simulink model "LinearSolver_System"  (R2021a)
settings: Solver=VariableStepAuto  StartTime=0.0  StopTime=1000  RelTol=1e-3
undefined symbols (not defined in the file or in its folder): AXI4, Lite
libraries: hdlBasic x415, xbsIndex_r4 x1
(part 3 of 4)

== system LinearSolver_System/Rotation4 ==
  y_in : Inport
  theta_in : Inport  Port=2
  rst : Inport  Port=3
  R_in : Inport  Port=4
  Constant3 : hdlBasic/Constant  const=0.0  gui_display_data_type=Fixed-point  arith_type=Signed (2's comp)  n_bits=16  bin_pt=13  preci_type=Single  exp_width=8  frac_width=24  explicit_period=off  period=1  XmcBlockStatus=1  maskContainerNames=tabcontainer1  block_type=constant  block_config=sysgen:Constant_config
  Constant4 : hdlBasic/Constant  const=1.0  gui_display_data_type=Boolean  arith_type=Boolean  n_bits=16  bin_pt=14  preci_type=Single  exp_width=8  frac_width=24  explicit_period=off  period=1  XmcBlockStatus=1  maskContainerNames=tabcontainer1  block_type=constant  block_config=sysgen:Constant_config
  Constant5 : hdlBasic/Constant  const=0  gui_display_data_type=Boolean  arith_type=Boolean  n_bits=16  bin_pt=14  preci_type=Single  exp_width=8  frac_width=24  explicit_period=off  period=1  XmcBlockStatus=1  maskContainerNames=tabcontainer1  block_type=constant  block_config=sysgen:Constant_config
  Constant6 : hdlBasic/Constant  const=0  gui_display_data_type=Boolean  arith_type=Boolean  n_bits=16  bin_pt=13  preci_type=Single  exp_width=8  frac_width=24  explicit_period=off  period=1  XmcBlockStatus=1  maskContainerNames=tabcontainer1  block_type=constant  block_config=sysgen:Constant_config
  Constant7 : hdlBasic/Constant  const=0.0  gui_display_data_type=Fixed-point  arith_type=Signed (2's comp)  n_bits=16  bin_pt=0  preci_type=Single  exp_width=8  frac_width=24  explicit_period=off  period=1  XmcBlockStatus=1  maskContainerNames=tabcontainer1  block_type=constant  block_config=sysgen:Constant_config
  Delay1 : hdlBasic/Delay  rst=off  en=off  latency=42  reg_retiming=off  XmcBlockStatus=1  maskContainerNames=group1  block_type=delay  block_config=sysgen:Delay_config
  Delay5 : hdlBasic/Delay  rst=off  en=off  latency=42  reg_retiming=off  XmcBlockStatus=1  maskContainerNames=group1  block_type=delay  block_config=sysgen:Delay_config
  Mux : hdlBasic/Mux  inputs=2  en=off  latency=0  precision=Full  arith_type=Unsigned  n_bits=16  bin_pt=14  quantization=Truncate  overflow=Wrap  XmcBlockStatus=1  maskContainerNames=tabcontainer1  block_type=mux  block_config=sysgen:Mux_config
  Mux2 : hdlBasic/Mux  inputs=2  en=off  latency=0  precision=Full  arith_type=Unsigned  n_bits=16  bin_pt=14  quantization=Truncate  overflow=Wrap  XmcBlockStatus=1  maskContainerNames=tabcontainer1  block_type=mux  block_config=sysgen:Mux_config
  Register : hdlBasic/Register  init=0  rst=on  en=off  XmcBlockStatus=1  maskContainerNames=tabcontainer1  block_type=register  block_config=sysgen:Register_config
  Scope6 : Scope
  Terminator{1..6} (6 alike) : Terminator
  Vitis HLS2 : hdlBasic/Vitis HLS  anytable='..\Vitis_HLS\project6_final_hls_mc\solution1_without_back_substitution'  fast_sim=off  display_datatype=off  rate_propagation_method=Simulink system period  model_file_path=''  latency=1  block_type=vitis_hls
      settings: infoedit=This block allows including C,C++ and SystemC source files in System Generator for DSP designs.
  theta_out : Outport
  y_out : Outport  Port=2
  x_out : Outport  Port=3
  sel_out : Outport  Port=4
  R_out : Outport  Port=5
  rst_out : Outport  Port=6
  wires:
  Mux/1 -> Mux2/3, Register/1
  Vitis HLS2/4 -> Mux/3, x_out/1
  y_in/1 -> Vitis HLS2/5
  Constant3/1 -> Mux/2
  Vitis HLS2/5 -> sel_out/1, Mux/1
  Vitis HLS2/6 -> y_out/1
  rst/1 -> Delay1/1, Mux2/1, Register/2
  Register/1 -> Vitis HLS2/4
  Constant6/1 -> Vitis HLS2/3
  Constant7/1 -> Vitis HLS2/7
  Constant4/1 -> Vitis HLS2/2
  Constant5/1 -> Vitis HLS2/1
  Vitis HLS2/3 -> Terminator6/1
  Vitis HLS2/2 -> Terminator1/1
  Vitis HLS2/1 -> Terminator3/1
  Vitis HLS2/8 -> Terminator5/1
  Vitis HLS2/7 -> Terminator2/1
  Vitis HLS2/9 -> Terminator4/1
  Mux2/1 -> R_out/1, Scope6/1
  R_in/1 -> Mux2/2
  theta_in/1 -> Delay5/1
  Delay5/1 -> Vitis HLS2/6, theta_out/1
  Delay1/1 -> rst_out/1

== system LinearSolver_System/Rotation5 ==
  y_in : Inport
  theta_in : Inport  Port=2
  sel_in : Inport  Port=3
  rst : Inport  Port=4
  R_in : Inport  Port=5
  Constant3 : hdlBasic/Constant  const=0.0  gui_display_data_type=Fixed-point  arith_type=Signed (2's comp)  n_bits=16  bin_pt=13  preci_type=Single  exp_width=8  frac_width=24  explicit_period=off  period=1  XmcBlockStatus=1  maskContainerNames=tabcontainer1  block_type=constant  block_config=sysgen:Constant_config
  Constant4 : hdlBasic/Constant  const=1.0  gui_display_data_type=Boolean  arith_type=Boolean  n_bits=16  bin_pt=14  preci_type=Single  exp_width=8  frac_width=24  explicit_period=off  period=1  XmcBlockStatus=1  maskContainerNames=tabcontainer1  block_type=constant  block_config=sysgen:Constant_config
  Constant5 : hdlBasic/Constant  const=0  gui_display_data_type=Boolean  arith_type=Boolean  n_bits=16  bin_pt=14  preci_type=Single  exp_width=8  frac_width=24  explicit_period=off  period=1  XmcBlockStatus=1  maskContainerNames=tabcontainer1  block_type=constant  block_config=sysgen:Constant_config
  Constant6 : hdlBasic/Constant  const=0  gui_display_data_type=Boolean  arith_type=Boolean  n_bits=16  bin_pt=13  preci_type=Single  exp_width=8  frac_width=24  explicit_period=off  period=1  XmcBlockStatus=1  maskContainerNames=tabcontainer1  block_type=constant  block_config=sysgen:Constant_config
  Constant7 : hdlBasic/Constant  const=0.0  gui_display_data_type=Fixed-point  arith_type=Signed (2's comp)  n_bits=16  bin_pt=0  preci_type=Single  exp_width=8  frac_width=24  explicit_period=off  period=1  XmcBlockStatus=1  maskContainerNames=tabcontainer1  block_type=constant  block_config=sysgen:Constant_config
  Delay1 : hdlBasic/Delay  rst=off  en=off  latency=42  reg_retiming=off  XmcBlockStatus=1  maskContainerNames=group1  block_type=delay  block_config=sysgen:Delay_config
  Delay2 : hdlBasic/Delay  rst=off  en=off  latency=43  reg_retiming=off  XmcBlockStatus=1  maskContainerNames=group1  block_type=delay  block_config=sysgen:Delay_config
  Delay5 : hdlBasic/Delay  rst=off  en=off  latency=42  reg_retiming=off  XmcBlockStatus=1  maskContainerNames=group1  block_type=delay  block_config=sysgen:Delay_config
  Mux : hdlBasic/Mux  inputs=2  en=off  latency=0  precision=Full  arith_type=Unsigned  n_bits=16  bin_pt=14  quantization=Truncate  overflow=Wrap  XmcBlockStatus=1  maskContainerNames=tabcontainer1  block_type=mux  block_config=sysgen:Mux_config
  Mux2 : hdlBasic/Mux  inputs=2  en=off  latency=0  precision=Full  arith_type=Unsigned  n_bits=16  bin_pt=14  quantization=Truncate  overflow=Wrap  XmcBlockStatus=1  maskContainerNames=tabcontainer1  block_type=mux  block_config=sysgen:Mux_config
  Register : hdlBasic/Register  init=0  rst=on  en=off  XmcBlockStatus=1  maskContainerNames=tabcontainer1  block_type=register  block_config=sysgen:Register_config
  Scope6 : Scope
  Terminator{1..7} (7 alike) : Terminator
  Vitis HLS2 : hdlBasic/Vitis HLS  anytable='..\Vitis_HLS\project6_final_hls_mc\solution1_without_back_substitution'  fast_sim=off  display_datatype=off  rate_propagation_method=Simulink system period  model_file_path=''  latency=1  block_type=vitis_hls
      settings: infoedit=This block allows including C,C++ and SystemC source files in System Generator for DSP designs.
  theta_out : Outport
  y_out : Outport  Port=2
  x_out : Outport  Port=3
  sel_out : Outport  Port=4
  R_out : Outport  Port=5
  rst_out : Outport  Port=6
  wires:
  Mux/1 -> Mux2/3, Register/1
  Vitis HLS2/4 -> Mux/3, x_out/1
  y_in/1 -> Vitis HLS2/5
  Constant3/1 -> Mux/2
  Vitis HLS2/6 -> y_out/1
  theta_in/1 -> Delay5/1
  sel_in/1 -> Delay2/1
  Register/1 -> Vitis HLS2/4
  Constant6/1 -> Vitis HLS2/3
  Constant7/1 -> Vitis HLS2/7
  Constant4/1 -> Vitis HLS2/2
  Constant5/1 -> Vitis HLS2/1
  Vitis HLS2/2 -> Terminator1/1
  Vitis HLS2/1 -> Terminator3/1
  Vitis HLS2/3 -> Terminator2/1
  Vitis HLS2/5 -> Terminator4/1
  Vitis HLS2/7 -> Terminator5/1
  Vitis HLS2/8 -> Terminator6/1
  Vitis HLS2/9 -> Terminator7/1
  Delay2/1 -> Mux/1, sel_out/1
  Mux2/1 -> R_out/1, Scope6/1
  R_in/1 -> Mux2/2
  Delay5/1 -> theta_out/1, Vitis HLS2/6
  Delay1/1 -> rst_out/1
  rst/1 -> Mux2/1, Register/2, Delay1/1

== system LinearSolver_System/Rotation6 ==
  y_in : Inport
  theta_in : Inport  Port=2
  sel_in : Inport  Port=3
  rst : Inport  Port=4
  R_in : Inport  Port=5
  Constant3 : hdlBasic/Constant  const=0.0  gui_display_data_type=Fixed-point  arith_type=Signed (2's comp)  n_bits=16  bin_pt=13  preci_type=Single  exp_width=8  frac_width=24  explicit_period=off  period=1  XmcBlockStatus=1  maskContainerNames=tabcontainer1  block_type=constant  block_config=sysgen:Constant_config
  Constant4 : hdlBasic/Constant  const=1.0  gui_display_data_type=Boolean  arith_type=Boolean  n_bits=16  bin_pt=14  preci_type=Single  exp_width=8  frac_width=24  explicit_period=off  period=1  XmcBlockStatus=1  maskContainerNames=tabcontainer1  block_type=constant  block_config=sysgen:Constant_config
  Constant5 : hdlBasic/Constant  const=0  gui_display_data_type=Boolean  arith_type=Boolean  n_bits=16  bin_pt=14  preci_type=Single  exp_width=8  frac_width=24  explicit_period=off  period=1  XmcBlockStatus=1  maskContainerNames=tabcontainer1  block_type=constant  block_config=sysgen:Constant_config
  Constant6 : hdlBasic/Constant  const=0  gui_display_data_type=Boolean  arith_type=Boolean  n_bits=16  bin_pt=13  preci_type=Single  exp_width=8  frac_width=24  explicit_period=off  period=1  XmcBlockStatus=1  maskContainerNames=tabcontainer1  block_type=constant  block_config=sysgen:Constant_config
  Constant7 : hdlBasic/Constant  const=0.0  gui_display_data_type=Fixed-point  arith_type=Signed (2's comp)  n_bits=16  bin_pt=0  preci_type=Single  exp_width=8  frac_width=24  explicit_period=off  period=1  XmcBlockStatus=1  maskContainerNames=tabcontainer1  block_type=constant  block_config=sysgen:Constant_config
  Delay2 : hdlBasic/Delay  rst=off  en=off  latency=43  reg_retiming=off  XmcBlockStatus=1  maskContainerNames=group1  block_type=delay  block_config=sysgen:Delay_config
  Delay5 : hdlBasic/Delay  rst=off  en=off  latency=0  reg_retiming=off  XmcBlockStatus=1  maskContainerNames=group1  block_type=delay  block_config=sysgen:Delay_config
  Mux : hdlBasic/Mux  inputs=2  en=off  latency=0  precision=Full  arith_type=Unsigned  n_bits=16  bin_pt=14  quantization=Truncate  overflow=Wrap  XmcBlockStatus=1  maskContainerNames=tabcontainer1  block_type=mux  block_config=sysgen:Mux_config
  Mux2 : hdlBasic/Mux  inputs=2  en=off  latency=0  precision=Full  arith_type=Unsigned  n_bits=16  bin_pt=14  quantization=Truncate  overflow=Wrap  XmcBlockStatus=1  maskContainerNames=tabcontainer1  block_type=mux  block_config=sysgen:Mux_config
  Register : hdlBasic/Register  init=0  rst=on  en=off  XmcBlockStatus=1  maskContainerNames=tabcontainer1  block_type=register  block_config=sysgen:Register_config
  Scope6 : Scope
  Terminator{1..7} (7 alike) : Terminator
  Vitis HLS2 : hdlBasic/Vitis HLS  anytable='..\Vitis_HLS\project6_final_hls_mc\solution1_without_back_substitution'  fast_sim=off  display_datatype=off  rate_propagation_method=Simulink system period  model_file_path=''  latency=1  block_type=vitis_hls
      settings: infoedit=This block allows including C,C++ and SystemC source files in System Generator for DSP designs.
  theta_out : Outport
  y_out : Outport  Port=2
  x_out : Outport  Port=3
  sel_out : Outport  Port=4
  R_out : Outport  Port=5
  wires:
  Vitis HLS2/4 -> x_out/1, Mux/3
  y_in/1 -> Vitis HLS2/5
  Constant3/1 -> Mux/2
  Vitis HLS2/6 -> y_out/1
  theta_in/1 -> Delay5/1
  sel_in/1 -> Delay2/1
  rst/1 -> Mux2/1, Register/2
  Register/1 -> Vitis HLS2/4
  Mux/1 -> Mux2/3, Register/1
  Constant6/1 -> Vitis HLS2/3
  Constant7/1 -> Vitis HLS2/7
  Constant4/1 -> Vitis HLS2/2
  Constant5/1 -> Vitis HLS2/1
  Vitis HLS2/9 -> Terminator7/1
  Vitis HLS2/8 -> Terminator6/1
  Vitis HLS2/7 -> Terminator5/1
  Vitis HLS2/5 -> Terminator4/1
  Vitis HLS2/3 -> Terminator2/1
  Vitis HLS2/2 -> Terminator1/1
  Vitis HLS2/1 -> Terminator3/1
  R_in/1 -> Mux2/2
  Mux2/1 -> R_out/1, Scope6/1
  Delay5/1 -> theta_out/1, Vitis HLS2/6
  Delay2/1 -> Mux/1, sel_out/1

== system LinearSolver_System/Rotation7 ==
  y_in : Inport
  theta_in : Inport  Port=2
  rst : Inport  Port=3
  Constant1 : hdlBasic/Constant  const=0.0  gui_display_data_type=Fixed-point  arith_type=Signed (2's comp)  n_bits=16  bin_pt=13  preci_type=Single  exp_width=8  frac_width=24  explicit_period=off  period=1  XmcBlockStatus=1  maskContainerNames=tabcontainer1  block_type=constant  block_config=sysgen:Constant_config
  Constant3 : hdlBasic/Constant  const=0.0  gui_display_data_type=Fixed-point  arith_type=Signed (2's comp)  n_bits=16  bin_pt=13  preci_type=Single  exp_width=8  frac_width=24  explicit_period=off  period=1  XmcBlockStatus=1  maskContainerNames=tabcontainer1  block_type=constant  block_config=sysgen:Constant_config
  Constant4 : hdlBasic/Constant  const=1.0  gui_display_data_type=Boolean  arith_type=Boolean  n_bits=16  bin_pt=14  preci_type=Single  exp_width=8  frac_width=24  explicit_period=off  period=1  XmcBlockStatus=1  maskContainerNames=tabcontainer1  block_type=constant  block_config=sysgen:Constant_config
  Constant5 : hdlBasic/Constant  const=0  gui_display_data_type=Boolean  arith_type=Boolean  n_bits=16  bin_pt=14  preci_type=Single  exp_width=8  frac_width=24  explicit_period=off  period=1  XmcBlockStatus=1  maskContainerNames=tabcontainer1  block_type=constant  block_config=sysgen:Constant_config
  Constant6 : hdlBasic/Constant  const=0  gui_display_data_type=Boolean  arith_type=Boolean  n_bits=16  bin_pt=13  preci_type=Single  exp_width=8  frac_width=24  explicit_period=off  period=1  XmcBlockStatus=1  maskContainerNames=tabcontainer1  block_type=constant  block_config=sysgen:Constant_config
  Constant7 : hdlBasic/Constant  const=0.0  gui_display_data_type=Fixed-point  arith_type=Signed (2's comp)  n_bits=16  bin_pt=0  preci_type=Single  exp_width=8  frac_width=24  explicit_period=off  period=1  XmcBlockStatus=1  maskContainerNames=tabcontainer1  block_type=constant  block_config=sysgen:Constant_config
  Delay1 : hdlBasic/Delay  rst=off  en=off  latency=42  reg_retiming=off  XmcBlockStatus=1  maskContainerNames=group1  block_type=delay  block_config=sysgen:Delay_config
  Delay5 : hdlBasic/Delay  rst=off  en=off  latency=42  reg_retiming=off  XmcBlockStatus=1  maskContainerNames=group1  block_type=delay  block_config=sysgen:Delay_config
  Mux : hdlBasic/Mux  inputs=2  en=off  latency=0  precision=Full  arith_type=Unsigned  n_bits=16  bin_pt=14  quantization=Truncate  overflow=Wrap  XmcBlockStatus=1  maskContainerNames=tabcontainer1  block_type=mux  block_config=sysgen:Mux_config
  Mux2 : hdlBasic/Mux  inputs=2  en=off  latency=0  precision=Full  arith_type=Unsigned  n_bits=16  bin_pt=14  quantization=Truncate  overflow=Wrap  XmcBlockStatus=1  maskContainerNames=tabcontainer1  block_type=mux  block_config=sysgen:Mux_config
  Register : hdlBasic/Register  init=0  rst=on  en=off  XmcBlockStatus=1  maskContainerNames=tabcontainer1  block_type=register  block_config=sysgen:Register_config
  Scope6 : Scope
  Terminator{1..6} (6 alike) : Terminator
  Vitis HLS2 : hdlBasic/Vitis HLS  anytable='..\Vitis_HLS\project6_final_hls_mc\solution1_without_back_substitution'  fast_sim=off  display_datatype=off  rate_propagation_method=Simulink system period  model_file_path=''  latency=1  block_type=vitis_hls
      settings: infoedit=This block allows including C,C++ and SystemC source files in System Generator for DSP designs.
  theta_out : Outport
  y_out : Outport  Port=2
  x_out : Outport  Port=3
  sel_out : Outport  Port=4
  Q_out : Outport  Port=5
  rst_out : Outport  Port=6
  wires:
  Vitis HLS2/4 -> x_out/1, Mux/3
  y_in/1 -> Vitis HLS2/5
  Constant3/1 -> Mux/2
  Vitis HLS2/5 -> Mux/1, sel_out/1
  Vitis HLS2/6 -> y_out/1
  rst/1 -> Delay1/1, Register/2, Mux2/1
  Register/1 -> Vitis HLS2/4
  Constant6/1 -> Vitis HLS2/3
  Constant7/1 -> Vitis HLS2/7
  Constant4/1 -> Vitis HLS2/2
  Constant5/1 -> Vitis HLS2/1
  Vitis HLS2/7 -> Terminator2/1
  Vitis HLS2/8 -> Terminator5/1
  Vitis HLS2/9 -> Terminator4/1
  Vitis HLS2/3 -> Terminator6/1
  Vitis HLS2/2 -> Terminator1/1
  Vitis HLS2/1 -> Terminator3/1
  Mux/1 -> Mux2/3, Register/1
  Mux2/1 -> Q_out/1, Scope6/1
  Constant1/1 -> Mux2/2
  Delay5/1 -> Vitis HLS2/6, theta_out/1
  theta_in/1 -> Delay5/1
  Delay1/1 -> rst_out/1

== system LinearSolver_System/Rotation8 ==
  y_in : Inport
  theta_in : Inport  Port=2
  sel_in : Inport  Port=3
  rst : Inport  Port=4
  Constant1 : hdlBasic/Constant  const=0.0  gui_display_data_type=Fixed-point  arith_type=Signed (2's comp)  n_bits=16  bin_pt=13  preci_type=Single  exp_width=8  frac_width=24  explicit_period=off  period=1  XmcBlockStatus=1  maskContainerNames=tabcontainer1  block_type=constant  block_config=sysgen:Constant_config
  Constant3 : hdlBasic/Constant  const=0.0  gui_display_data_type=Fixed-point  arith_type=Signed (2's comp)  n_bits=16  bin_pt=13  preci_type=Single  exp_width=8  frac_width=24  explicit_period=off  period=1  XmcBlockStatus=1  maskContainerNames=tabcontainer1  block_type=constant  block_config=sysgen:Constant_config
  Constant4 : hdlBasic/Constant  const=1.0  gui_display_data_type=Boolean  arith_type=Boolean  n_bits=16  bin_pt=14  preci_type=Single  exp_width=8  frac_width=24  explicit_period=off  period=1  XmcBlockStatus=1  maskContainerNames=tabcontainer1  block_type=constant  block_config=sysgen:Constant_config
  Constant5 : hdlBasic/Constant  const=0  gui_display_data_type=Boolean  arith_type=Boolean  n_bits=16  bin_pt=14  preci_type=Single  exp_width=8  frac_width=24  explicit_period=off  period=1  XmcBlockStatus=1  maskContainerNames=tabcontainer1  block_type=constant  block_config=sysgen:Constant_config
  Constant6 : hdlBasic/Constant  const=0  gui_display_data_type=Boolean  arith_type=Boolean  n_bits=16  bin_pt=13  preci_type=Single  exp_width=8  frac_width=24  explicit_period=off  period=1  XmcBlockStatus=1  maskContainerNames=tabcontainer1  block_type=constant  block_config=sysgen:Constant_config
  Constant7 : hdlBasic/Constant  const=0.0  gui_display_data_type=Fixed-point  arith_type=Signed (2's comp)  n_bits=16  bin_pt=0  preci_type=Single  exp_width=8  frac_width=24  explicit_period=off  period=1  XmcBlockStatus=1  maskContainerNames=tabcontainer1  block_type=constant  block_config=sysgen:Constant_config
  Delay1 : hdlBasic/Delay  rst=off  en=off  latency=42  reg_retiming=off  XmcBlockStatus=1  maskContainerNames=group1  block_type=delay  block_config=sysgen:Delay_config
  Delay2 : hdlBasic/Delay  rst=off  en=off  latency=43  reg_retiming=off  XmcBlockStatus=1  maskContainerNames=group1  block_type=delay  block_config=sysgen:Delay_config
  Delay5 : hdlBasic/Delay  rst=off  en=off  latency=42  reg_retiming=off  XmcBlockStatus=1  maskContainerNames=group1  block_type=delay  block_config=sysgen:Delay_config
  Mux : hdlBasic/Mux  inputs=2  en=off  latency=0  precision=Full  arith_type=Unsigned  n_bits=16  bin_pt=14  quantization=Truncate  overflow=Wrap  XmcBlockStatus=1  maskContainerNames=tabcontainer1  block_type=mux  block_config=sysgen:Mux_config
  Mux2 : hdlBasic/Mux  inputs=2  en=off  latency=0  precision=Full  arith_type=Unsigned  n_bits=16  bin_pt=14  quantization=Truncate  overflow=Wrap  XmcBlockStatus=1  maskContainerNames=tabcontainer1  block_type=mux  block_config=sysgen:Mux_config
  Register : hdlBasic/Register  init=0  rst=on  en=off  XmcBlockStatus=1  maskContainerNames=tabcontainer1  block_type=register  block_config=sysgen:Register_config
  Scope6 : Scope
  Terminator{1..7} (7 alike) : Terminator
  Vitis HLS2 : hdlBasic/Vitis HLS  anytable='..\Vitis_HLS\project6_final_hls_mc\solution1_without_back_substitution'  fast_sim=off  display_datatype=off  rate_propagation_method=Simulink system period  model_file_path=''  latency=1  block_type=vitis_hls
      settings: infoedit=This block allows including C,C++ and SystemC source files in System Generator for DSP designs.
  theta_out : Outport
  y_out : Outport  Port=2
  x_out : Outport  Port=3
  sel_out : Outport  Port=4
  Q_out : Outport  Port=5
  rst_out : Outport  Port=6
  wires:
  Mux/1 -> Mux2/3, Register/1
  Vitis HLS2/4 -> x_out/1, Mux/3
  y_in/1 -> Vitis HLS2/5
  Constant3/1 -> Mux/2
  Vitis HLS2/6 -> y_out/1
  theta_in/1 -> Delay5/1
  Register/1 -> Vitis HLS2/4
  rst/1 -> Delay1/1, Mux2/1, Register/2
  Constant6/1 -> Vitis HLS2/3
  Constant7/1 -> Vitis HLS2/7
  Constant4/1 -> Vitis HLS2/2
  Constant5/1 -> Vitis HLS2/1
  Vitis HLS2/1 -> Terminator3/1
  Vitis HLS2/2 -> Terminator1/1
  Vitis HLS2/3 -> Terminator2/1
  Vitis HLS2/5 -> Terminator4/1
  Vitis HLS2/7 -> Terminator5/1
  Vitis HLS2/8 -> Terminator6/1
  Vitis HLS2/9 -> Terminator7/1
  sel_in/1 -> Delay2/1
  Delay2/1 -> Mux/1, sel_out/1
  Mux2/1 -> Q_out/1, Scope6/1
  Constant1/1 -> Mux2/2
  Delay5/1 -> theta_out/1, Vitis HLS2/6
  Delay1/1 -> rst_out/1

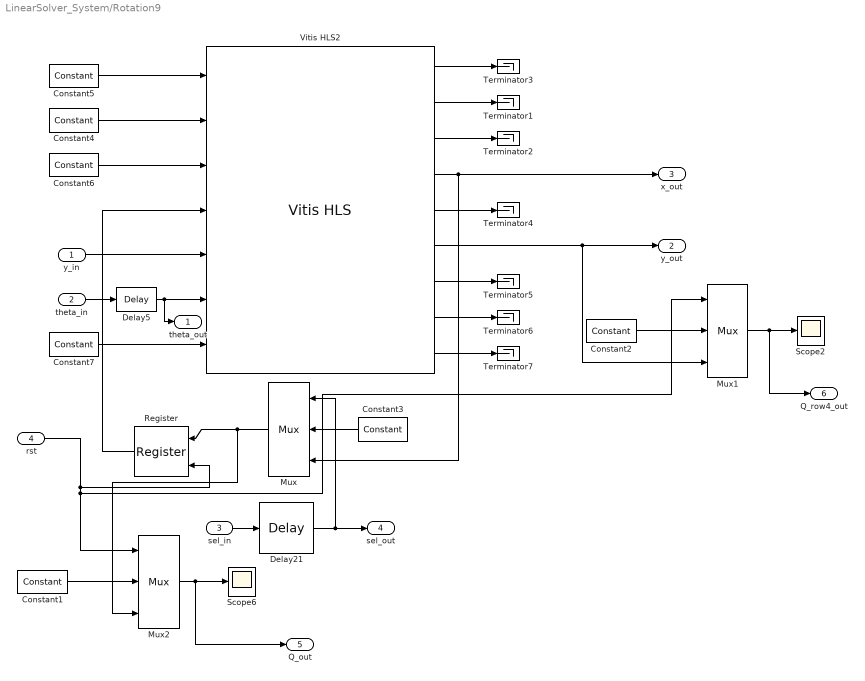
== system LinearSolver_System/Rotation9 ==
  y_in : Inport
  theta_in : Inport  Port=2
  sel_in : Inport  Port=3
  rst : Inport  Port=4
  Constant1 : hdlBasic/Constant  const=0.0  gui_display_data_type=Fixed-point  arith_type=Signed (2's comp)  n_bits=16  bin_pt=13  preci_type=Single  exp_width=8  frac_width=24  explicit_period=off  period=1  XmcBlockStatus=1  maskContainerNames=tabcontainer1  block_type=constant  block_config=sysgen:Constant_config
  Constant2 : hdlBasic/Constant  const=0.0  gui_display_data_type=Fixed-point  arith_type=Signed (2's comp)  n_bits=16  bin_pt=13  preci_type=Single  exp_width=8  frac_width=24  explicit_period=off  period=1  XmcBlockStatus=1  maskContainerNames=tabcontainer1  block_type=constant  block_config=sysgen:Constant_config
  Constant3 : hdlBasic/Constant  const=0.0  gui_display_data_type=Fixed-point  arith_type=Signed (2's comp)  n_bits=16  bin_pt=13  preci_type=Single  exp_width=8  frac_width=24  explicit_period=off  period=1  XmcBlockStatus=1  maskContainerNames=tabcontainer1  block_type=constant  block_config=sysgen:Constant_config
  Constant4 : hdlBasic/Constant  const=1.0  gui_display_data_type=Boolean  arith_type=Boolean  n_bits=16  bin_pt=14  preci_type=Single  exp_width=8  frac_width=24  explicit_period=off  period=1  XmcBlockStatus=1  maskContainerNames=tabcontainer1  block_type=constant  block_config=sysgen:Constant_config
  Constant5 : hdlBasic/Constant  const=0  gui_display_data_type=Boolean  arith_type=Boolean  n_bits=16  bin_pt=14  preci_type=Single  exp_width=8  frac_width=24  explicit_period=off  period=1  XmcBlockStatus=1  maskContainerNames=tabcontainer1  block_type=constant  block_config=sysgen:Constant_config
  Constant6 : hdlBasic/Constant  const=0  gui_display_data_type=Boolean  arith_type=Boolean  n_bits=16  bin_pt=13  preci_type=Single  exp_width=8  frac_width=24  explicit_period=off  period=1  XmcBlockStatus=1  maskContainerNames=tabcontainer1  block_type=constant  block_config=sysgen:Constant_config
  Constant7 : hdlBasic/Constant  const=0.0  gui_display_data_type=Fixed-point  arith_type=Signed (2's comp)  n_bits=16  bin_pt=0  preci_type=Single  exp_width=8  frac_width=24  explicit_period=off  period=1  XmcBlockStatus=1  maskContainerNames=tabcontainer1  block_type=constant  block_config=sysgen:Constant_config
  Delay21 : hdlBasic/Delay  rst=off  en=off  latency=43  reg_retiming=off  XmcBlockStatus=1  maskContainerNames=group1  block_type=delay  block_config=sysgen:Delay_config
  Delay5 : hdlBasic/Delay  rst=off  en=off  latency=42  reg_retiming=off  XmcBlockStatus=1  maskContainerNames=group1  block_type=delay  block_config=sysgen:Delay_config
  Mux : hdlBasic/Mux  inputs=2  en=off  latency=0  precision=Full  arith_type=Unsigned  n_bits=16  bin_pt=14  quantization=Truncate  overflow=Wrap  XmcBlockStatus=1  maskContainerNames=tabcontainer1  block_type=mux  block_config=sysgen:Mux_config
  Mux1 : hdlBasic/Mux  inputs=2  en=off  latency=0  precision=Full  arith_type=Unsigned  n_bits=16  bin_pt=14  quantization=Truncate  overflow=Wrap  XmcBlockStatus=1  maskContainerNames=tabcontainer1  block_type=mux  block_config=sysgen:Mux_config
  Mux2 : hdlBasic/Mux  inputs=2  en=off  latency=0  precision=Full  arith_type=Unsigned  n_bits=16  bin_pt=14  quantization=Truncate  overflow=Wrap  XmcBlockStatus=1  maskContainerNames=tabcontainer1  block_type=mux  block_config=sysgen:Mux_config
  Register : hdlBasic/Register  init=0  rst=on  en=off  XmcBlockStatus=1  maskContainerNames=tabcontainer1  block_type=register  block_config=sysgen:Register_config
  Scope2 : Scope
  Scope6 : Scope
  Terminator{1..7} (7 alike) : Terminator
  Vitis HLS2 : hdlBasic/Vitis HLS  anytable='..\Vitis_HLS\project6_final_hls_mc\solution1_without_back_substitution'  fast_sim=off  display_datatype=off  rate_propagation_method=Simulink system period  model_file_path=''  latency=1  block_type=vitis_hls
      settings: infoedit=This block allows including C,C++ and SystemC source files in System Generator for DSP designs.
  theta_out : Outport
  y_out : Outport  Port=2
  x_out : Outport  Port=3
  sel_out : Outport  Port=4
  Q_out : Outport  Port=5
  Q_row4_out : Outport  Port=6
  wires:
  Mux/1 -> Mux2/3, Register/1
  Vitis HLS2/4 -> Mux/3, x_out/1
  y_in/1 -> Vitis HLS2/5
  Constant3/1 -> Mux/2
  theta_in/1 -> Delay5/1
  sel_in/1 -> Delay21/1
  Register/1 -> Vitis HLS2/4
  rst/1 -> Mux1/1, Mux2/1, Register/2
  Delay21/1 -> sel_out/1, Mux/1
  Constant6/1 -> Vitis HLS2/3
  Constant7/1 -> Vitis HLS2/7
  Constant4/1 -> Vitis HLS2/2
  Constant5/1 -> Vitis HLS2/1
  Vitis HLS2/1 -> Terminator3/1
  Vitis HLS2/2 -> Terminator1/1
  Vitis HLS2/3 -> Terminator2/1
  Vitis HLS2/5 -> Terminator4/1
  Vitis HLS2/7 -> Terminator5/1
  Vitis HLS2/8 -> Terminator6/1
  Vitis HLS2/9 -> Terminator7/1
  Constant1/1 -> Mux2/2
  Mux1/1 -> Q_row4_out/1, Scope2/1
  Constant2/1 -> Mux1/2
  Vitis HLS2/6 -> Mux1/3, y_out/1
  Mux2/1 -> Q_out/1, Scope6/1
  Delay5/1 -> theta_out/1, Vitis HLS2/6

== system LinearSolver_System/Subsystem ==
  QT_row1_In : Inport
  rst_b_In : Inport  Port=2
  b_col_In : Inport  Port=3
  AddSub : hdlBasic/AddSub  mode=Addition  use_carryin=off  use_carryout=off  en=off  latency=0  precision=Full  arith_type=Unsigned  n_bits=16  bin_pt=14  quantization=Truncate  overflow=Wrap  use_behavioral_HDL=off  hw_selection=Fabric  pipelined=off  XmcBlockStatus=1  maskContainerNames=tabcontainer1  block_type=addsub  block_config=sysgen:Addsub_config
  AddSub1 : hdlBasic/AddSub  mode=Addition  use_carryin=off  use_carryout=off  en=off  latency=0  precision=Full  arith_type=Unsigned  n_bits=16  bin_pt=14  quantization=Truncate  overflow=Wrap  use_behavioral_HDL=off  hw_selection=Fabric  pipelined=off  XmcBlockStatus=1  maskContainerNames=tabcontainer1  block_type=addsub  block_config=sysgen:Addsub_config
  AddSub2 : hdlBasic/AddSub  mode=Addition  use_carryin=off  use_carryout=off  en=off  latency=0  precision=Full  arith_type=Unsigned  n_bits=16  bin_pt=14  quantization=Truncate  overflow=Wrap  use_behavioral_HDL=off  hw_selection=Fabric  pipelined=off  XmcBlockStatus=1  maskContainerNames=tabcontainer1  block_type=addsub  block_config=sysgen:Addsub_config
  Delay{,1..6} (7 alike) : hdlBasic/Delay  rst=off  en=off  latency=42  reg_retiming=off  XmcBlockStatus=1  maskContainerNames=group1  block_type=delay  block_config=sysgen:Delay_config
  Init Boolean1 : hdlBasic/Constant  const=0  gui_display_data_type=Fixed-point  arith_type=Signed (2's comp)  n_bits=16  bin_pt=14  preci_type=Single  exp_width=8  frac_width=24  explicit_period=off  period=1  XmcBlockStatus=1  maskContainerNames=tabcontainer1  block_type=constant  block_config=sysgen:Constant_config
  Mult : hdlBasic/Mult  precision=Full  arith_type="Signed  (2's comp)"  n_bits=16  bin_pt=14  quantization=Truncate  overflow=Wrap  en=off  latency=0  use_behavioral_HDL=off  opt=Speed  use_embedded=on  optimum_pipeline=off  pipeline=on  use_rpm=on  placement_style=Triangular  XmcBlockStatus=1  maskContainerNames=group1  block_type=mult  block_config=sysgen:Mult_config
  Mux2 : hdlBasic/Mux  inputs=2  en=off  latency=0  precision=Full  arith_type=Unsigned  n_bits=16  bin_pt=14  quantization=Truncate  overflow=Wrap  XmcBlockStatus=1  maskContainerNames=tabcontainer1  block_type=mux  block_config=sysgen:Mux_config
  Scope{1..5,23} (6 alike) : Scope
  rst_b_out : Outport
  b_col_out : Outport  Port=2
  y_out : Outport  Port=3
  wires:
  QT_row1_In/1 -> Mult/1
  b_col_In/1 -> b_col_out/1, Mult/2
  rst_b_In/1 -> Delay1/1
  Delay1/1 -> Delay2/1
  Delay3/1 -> Delay4/1, AddSub1/1
  Mult/1 -> AddSub/2, Scope23/1, Delay/1
  AddSub1/1 -> Scope1/1, AddSub2/2
  Delay4/1 -> AddSub2/1
  Delay/1 -> AddSub/1, Delay3/1
  AddSub/1 -> AddSub1/2, Scope4/1
  AddSub2/1 -> Mux2/3, Scope3/1
  Delay2/1 -> Delay5/1
  Delay5/1 -> Delay6/1
  Init Boolean1/1 -> Mux2/2
  Delay6/1 -> rst_b_out/1, Scope2/1, Mux2/1
  Mux2/1 -> y_out/1, Scope5/1

== system LinearSolver_System/Subsystem1 ==
  QT_row2_In : Inport
  rst_b_In : Inport  Port=2
  b_col_In : Inport  Port=3
  Qb_In : Inport  Port=4
  AddSub : hdlBasic/AddSub  mode=Addition  use_carryin=off  use_carryout=off  en=off  latency=0  precision=Full  arith_type=Unsigned  n_bits=16  bin_pt=14  quantization=Truncate  overflow=Wrap  use_behavioral_HDL=off  hw_selection=Fabric  pipelined=off  XmcBlockStatus=1  maskContainerNames=tabcontainer1  block_type=addsub  block_config=sysgen:Addsub_config
  AddSub1 : hdlBasic/AddSub  mode=Addition  use_carryin=off  use_carryout=off  en=off  latency=0  precision=Full  arith_type=Unsigned  n_bits=16  bin_pt=14  quantization=Truncate  overflow=Wrap  use_behavioral_HDL=off  hw_selection=Fabric  pipelined=off  XmcBlockStatus=1  maskContainerNames=tabcontainer1  block_type=addsub  block_config=sysgen:Addsub_config
  AddSub2 : hdlBasic/AddSub  mode=Addition  use_carryin=off  use_carryout=off  en=off  latency=0  precision=Full  arith_type=Unsigned  n_bits=16  bin_pt=14  quantization=Truncate  overflow=Wrap  use_behavioral_HDL=off  hw_selection=Fabric  pipelined=off  XmcBlockStatus=1  maskContainerNames=tabcontainer1  block_type=addsub  block_config=sysgen:Addsub_config
  Delay{,1,3..5} (5 alike) : hdlBasic/Delay  rst=off  en=off  latency=42  reg_retiming=off  XmcBlockStatus=1  maskContainerNames=group1  block_type=delay  block_config=sysgen:Delay_config
  Mult : hdlBasic/Mult  precision=Full  arith_type="Signed  (2's comp)"  n_bits=16  bin_pt=14  quantization=Truncate  overflow=Wrap  en=off  latency=0  use_behavioral_HDL=off  opt=Speed  use_embedded=on  optimum_pipeline=off  pipeline=on  use_rpm=on  placement_style=Triangular  XmcBlockStatus=1  maskContainerNames=group1  block_type=mult  block_config=sysgen:Mult_config
  Mux2 : hdlBasic/Mux  inputs=2  en=off  latency=0  precision=Full  arith_type=Unsigned  n_bits=16  bin_pt=14  quantization=Truncate  overflow=Wrap  XmcBlockStatus=1  maskContainerNames=tabcontainer1  block_type=mux  block_config=sysgen:Mux_config
  Negate11 : hdlBasic/Negate  precision=User Defined  arith_type="Signed  (2's comp)"  n_bits=16  bin_pt=13  quantization=Truncate  overflow=Wrap  en=off  latency=0  XmcBlockStatus=1  maskContainerNames=tabcontainer1  block_type=negate  block_config=sysgen:Negate_config
  Scope{1..5,23} (6 alike) : Scope
  rst_b_out : Outport
  b_col_out : Outport  Port=2
  y_out : Outport  Port=3
  wires:
  QT_row2_In/1 -> Mult/1
  b_col_In/1 -> Delay1/1
  rst_b_In/1 -> Delay5/1
  Delay1/1 -> b_col_out/1, Mult/2
  Delay5/1 -> rst_b_out/1, Scope2/1, Mux2/1
  Delay3/1 -> Delay4/1, AddSub1/1
  Delay/1 -> AddSub/1, Delay3/1
  AddSub/1 -> Scope4/1, AddSub1/2
  Mult/1 -> AddSub/2, Scope23/1, Delay/1
  AddSub1/1 -> Scope1/1, AddSub2/2
  AddSub2/1 -> Scope3/1, Negate11/1
  Mux2/1 -> y_out/1, Scope5/1
  Delay4/1 -> AddSub2/1
  Qb_In/1 -> Mux2/2
  Negate11/1 -> Mux2/3

== system LinearSolver_System/Subsystem2 ==
  QT_row3_In : Inport
  rst_b_In : Inport  Port=2
  b_col_In : Inport  Port=3
  Qb_In : Inport  Port=4
  AddSub : hdlBasic/AddSub  mode=Addition  use_carryin=off  use_carryout=off  en=off  latency=0  precision=Full  arith_type=Unsigned  n_bits=16  bin_pt=14  quantization=Truncate  overflow=Wrap  use_behavioral_HDL=off  hw_selection=Fabric  pipelined=off  XmcBlockStatus=1  maskContainerNames=tabcontainer1  block_type=addsub  block_config=sysgen:Addsub_config
  AddSub1 : hdlBasic/AddSub  mode=Addition  use_carryin=off  use_carryout=off  en=off  latency=0  precision=Full  arith_type=Unsigned  n_bits=16  bin_pt=14  quantization=Truncate  overflow=Wrap  use_behavioral_HDL=off  hw_selection=Fabric  pipelined=off  XmcBlockStatus=1  maskContainerNames=tabcontainer1  block_type=addsub  block_config=sysgen:Addsub_config
  AddSub2 : hdlBasic/AddSub  mode=Addition  use_carryin=off  use_carryout=off  en=off  latency=0  precision=Full  arith_type=Unsigned  n_bits=16  bin_pt=14  quantization=Truncate  overflow=Wrap  use_behavioral_HDL=off  hw_selection=Fabric  pipelined=off  XmcBlockStatus=1  maskContainerNames=tabcontainer1  block_type=addsub  block_config=sysgen:Addsub_config
  Delay{,1,3..5} (5 alike) : hdlBasic/Delay  rst=off  en=off  latency=42  reg_retiming=off  XmcBlockStatus=1  maskContainerNames=group1  block_type=delay  block_config=sysgen:Delay_config
  Mult : hdlBasic/Mult  precision=Full  arith_type="Signed  (2's comp)"  n_bits=16  bin_pt=14  quantization=Truncate  overflow=Wrap  en=off  latency=0  use_behavioral_HDL=off  opt=Speed  use_embedded=on  optimum_pipeline=off  pipeline=on  use_rpm=on  placement_style=Triangular  XmcBlockStatus=1  maskContainerNames=group1  block_type=mult  block_config=sysgen:Mult_config
  Mux2 : hdlBasic/Mux  inputs=2  en=off  latency=0  precision=Full  arith_type=Unsigned  n_bits=16  bin_pt=14  quantization=Truncate  overflow=Wrap  XmcBlockStatus=1  maskContainerNames=tabcontainer1  block_type=mux  block_config=sysgen:Mux_config
  Scope{1..5,23} (6 alike) : Scope
  rst_b_out : Outport
  b_col_out : Outport  Port=2
  y_out : Outport  Port=3
  wires:
  QT_row3_In/1 -> Mult/1
  b_col_In/1 -> Delay1/1
  rst_b_In/1 -> Delay5/1
  Delay1/1 -> b_col_out/1, Mult/2
  Delay5/1 -> rst_b_out/1, Scope2/1, Mux2/1
  Delay3/1 -> Delay4/1, AddSub1/1
  Delay/1 -> AddSub/1, Delay3/1
  AddSub/1 -> Scope4/1, AddSub1/2
  Mult/1 -> AddSub/2, Scope23/1, Delay/1
  AddSub1/1 -> Scope1/1, AddSub2/2
  AddSub2/1 -> Mux2/3, Scope3/1
  Mux2/1 -> y_out/1, Scope5/1
  Delay4/1 -> AddSub2/1
  Qb_In/1 -> Mux2/2

== system LinearSolver_System/Subsystem3 ==
  QT_row4_In : Inport
  rst_b_In : Inport  Port=2
  b_col_In : Inport  Port=3
  Qb_In : Inport  Port=4
  AddSub : hdlBasic/AddSub  mode=Addition  use_carryin=off  use_carryout=off  en=off  latency=0  precision=Full  arith_type=Unsigned  n_bits=16  bin_pt=14  quantization=Truncate  overflow=Wrap  use_behavioral_HDL=off  hw_selection=Fabric  pipelined=off  XmcBlockStatus=1  maskContainerNames=tabcontainer1  block_type=addsub  block_config=sysgen:Addsub_config
  AddSub1 : hdlBasic/AddSub  mode=Addition  use_carryin=off  use_carryout=off  en=off  latency=0  precision=Full  arith_type=Unsigned  n_bits=16  bin_pt=14  quantization=Truncate  overflow=Wrap  use_behavioral_HDL=off  hw_selection=Fabric  pipelined=off  XmcBlockStatus=1  maskContainerNames=tabcontainer1  block_type=addsub  block_config=sysgen:Addsub_config
  AddSub2 : hdlBasic/AddSub  mode=Addition  use_carryin=off  use_carryout=off  en=off  latency=0  precision=Full  arith_type=Unsigned  n_bits=16  bin_pt=14  quantization=Truncate  overflow=Wrap  use_behavioral_HDL=off  hw_selection=Fabric  pipelined=off  XmcBlockStatus=1  maskContainerNames=tabcontainer1  block_type=addsub  block_config=sysgen:Addsub_config
  Delay{,3..5} (4 alike) : hdlBasic/Delay  rst=off  en=off  latency=42  reg_retiming=off  XmcBlockStatus=1  maskContainerNames=group1  block_type=delay  block_config=sysgen:Delay_config
  Mult : hdlBasic/Mult  precision=Full  arith_type="Signed  (2's comp)"  n_bits=16  bin_pt=14  quantization=Truncate  overflow=Wrap  en=off  latency=0  use_behavioral_HDL=off  opt=Speed  use_embedded=on  optimum_pipeline=off  pipeline=on  use_rpm=on  placement_style=Triangular  XmcBlockStatus=1  maskContainerNames=group1  block_type=mult  block_config=sysgen:Mult_config
  Mux2 : hdlBasic/Mux  inputs=2  en=off  latency=0  precision=User Defined  arith_type="Signed  (2's comp)"  n_bits=16  bin_pt=13  quantization="Round  (unbiased: +/- Inf)"  overflow=Saturate  XmcBlockStatus=1  maskContainerNames=tabcontainer1  block_type=mux  block_config=sysgen:Mux_config
  Negate11 : hdlBasic/Negate  precision=User Defined  arith_type="Signed  (2's comp)"  n_bits=16  bin_pt=13  quantization=Truncate  overflow=Wrap  en=off  latency=42  XmcBlockStatus=1  maskContainerNames=tabcontainer1  block_type=negate  block_config=sysgen:Negate_config
  Scope{1..7,23} (8 alike) : Scope
  rst_b_out : Outport
  b_col_out : Outport  Port=2
  y_out : Outport  Port=3
  wires:
  QT_row4_In/1 -> Scope7/1, Mult/1
  rst_b_In/1 -> Delay5/1
  b_col_In/1 -> Scope6/1, b_col_out/1, Mult/2
  Delay5/1 -> rst_b_out/1, Scope2/1, Mux2/1
  Delay3/1 -> Delay4/1, AddSub1/1
  Delay/1 -> AddSub/1, Delay3/1
  AddSub/1 -> Scope4/1, AddSub1/2
  Mult/1 -> AddSub/2, Scope23/1, Delay/1
  AddSub1/1 -> Scope1/1, AddSub2/2
  Mux2/1 -> y_out/1, Scope5/1
  Delay4/1 -> AddSub2/1
  Qb_In/1 -> Mux2/2
  AddSub2/1 -> Negate11/1, Scope3/1
  Negate11/1 -> Mux2/3

== system LinearSolver_System/Subsystem4 ==
  note: 633th
  note: y4 / R44 = d
  R_in : Inport
  QTb_in : Inport  Port=2
  Constant{1..3,8} (4 alike) : hdlBasic/Constant  const=0.0  gui_display_data_type=Fixed-point  arith_type=Signed (2's comp)  n_bits=16  bin_pt=13  preci_type=Single  exp_width=8  frac_width=24  explicit_period=off  period=1  XmcBlockStatus=1  maskContainerNames=tabcontainer1  block_type=constant  block_config=sysgen:Constant_config
  Constant4 : hdlBasic/Constant  const=1.0  gui_display_data_type=Boolean  arith_type=Boolean  n_bits=16  bin_pt=14  preci_type=Single  exp_width=8  frac_width=24  explicit_period=off  period=1  XmcBlockStatus=1  maskContainerNames=tabcontainer1  block_type=constant  block_config=sysgen:Constant_config
  Constant5 : hdlBasic/Constant  const=0  gui_display_data_type=Boolean  arith_type=Boolean  n_bits=16  bin_pt=14  preci_type=Single  exp_width=8  frac_width=24  explicit_period=off  period=1  XmcBlockStatus=1  maskContainerNames=tabcontainer1  block_type=constant  block_config=sysgen:Constant_config
  Constant6 : hdlBasic/Constant  const=0  gui_display_data_type=Boolean  arith_type=Boolean  n_bits=16  bin_pt=13  preci_type=Single  exp_width=8  frac_width=24  explicit_period=off  period=1  XmcBlockStatus=1  maskContainerNames=tabcontainer1  block_type=constant  block_config=sysgen:Constant_config
  Constant7 : hdlBasic/Constant  const=0.0  gui_display_data_type=Fixed-point  arith_type=Signed (2's comp)  n_bits=16  bin_pt=0  preci_type=Single  exp_width=8  frac_width=24  explicit_period=off  period=1  XmcBlockStatus=1  maskContainerNames=tabcontainer1  block_type=constant  block_config=sysgen:Constant_config
  Mux2 : hdlBasic/Mux  inputs=2  en=off  latency=0  precision=User Defined  arith_type="Signed  (2's comp)"  n_bits=16  bin_pt=13  quantization="Round  (unbiased: +/- Inf)"  overflow=Saturate  XmcBlockStatus=1  maskContainerNames=tabcontainer1  block_type=mux  block_config=sysgen:Mux_config
  Scope1 : Scope
  Terminator{1..3,5..6,8..11} (9 alike) : Terminator
  Vitis HLS2 : hdlBasic/Vitis HLS  anytable='..\Vitis_HLS\project6_final_hls_mc\solution2_add_back_substitution'  fast_sim=off  display_datatype=off  rate_propagation_method=Simulink system period  model_file_path=''  latency=1  block_type=vitis_hls
      settings: infoedit=This block allows including C,C++ and SystemC source files in System Generator for DSP designs.
  X_out : Outport
  wires:
  Constant4/1 -> Vitis HLS2/2
  Vitis HLS2/11 -> Mux2/1
  Vitis HLS2/4 -> Terminator10/1
  Constant2/1 -> Vitis HLS2/5
  Constant3/1 -> Vitis HLS2/6
  Constant5/1 -> Vitis HLS2/1
  Vitis HLS2/2 -> Terminator1/1
  Vitis HLS2/8 -> Terminator8/1
  Vitis HLS2/9 -> Terminator9/1
  Vitis HLS2/1 -> Terminator3/1
  Constant1/1 -> Vitis HLS2/4
  Constant6/1 -> Vitis HLS2/3
  Constant7/1 -> Vitis HLS2/7
  Vitis HLS2/3 -> Terminator2/1
  Vitis HLS2/5 -> Terminator5/1
  Vitis HLS2/7 -> Terminator6/1
  Vitis HLS2/10 -> Mux2/3
  Vitis HLS2/6 -> Terminator11/1
  QTb_in/1 -> Vitis HLS2/9
  R_in/1 -> Vitis HLS2/8
  Constant8/1 -> Mux2/2
  Mux2/1 -> Scope1/1, X_out/1

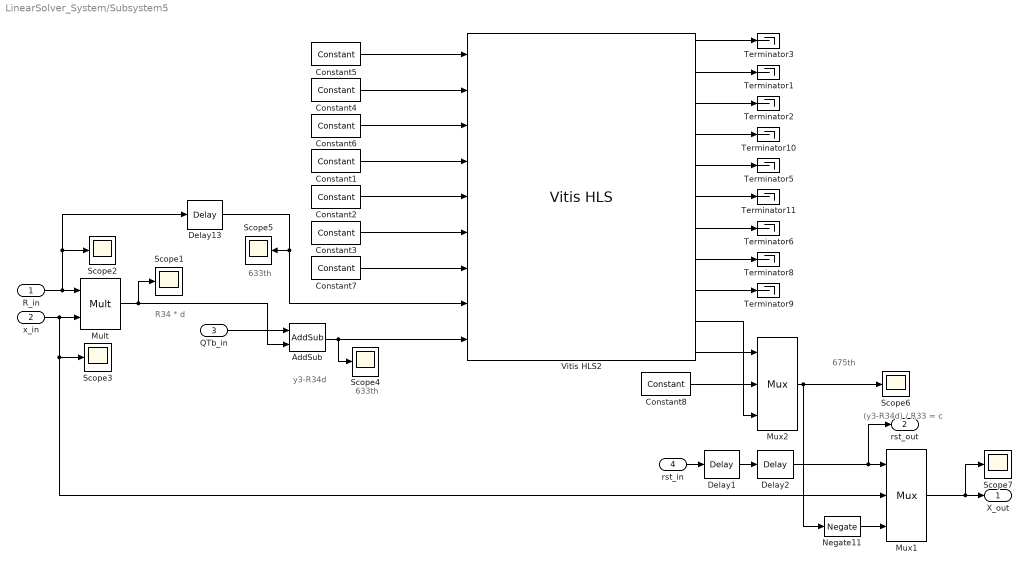
== system LinearSolver_System/Subsystem5 ==
  note: 675th
  note: R34 * d
  note: y3-R34d
  note: 633th
  note: 633th
  note: (y3-R34d) / R33 = c
  R_in : Inport
  x_in : Inport  Port=2
  QTb_in : Inport  Port=3
  rst_in : Inport  Port=4
  AddSub : hdlBasic/AddSub  mode=Subtraction  use_carryin=off  use_carryout=off  en=off  latency=0  precision=User Defined  arith_type="Signed  (2's comp)"  n_bits=16  bin_pt=13  quantization="Round  (unbiased: +/- Inf)"  overflow=Saturate  use_behavioral_HDL=off  hw_selection=Fabric  pipelined=off  XmcBlockStatus=1  maskContainerNames=tabcontainer1  block_type=addsub  block_config=sysgen:Addsub_config
  Constant{1..3,8} (4 alike) : hdlBasic/Constant  const=0.0  gui_display_data_type=Fixed-point  arith_type=Signed (2's comp)  n_bits=16  bin_pt=13  preci_type=Single  exp_width=8  frac_width=24  explicit_period=off  period=1  XmcBlockStatus=1  maskContainerNames=tabcontainer1  block_type=constant  block_config=sysgen:Constant_config
  Constant4 : hdlBasic/Constant  const=1.0  gui_display_data_type=Boolean  arith_type=Boolean  n_bits=16  bin_pt=14  preci_type=Single  exp_width=8  frac_width=24  explicit_period=off  period=1  XmcBlockStatus=1  maskContainerNames=tabcontainer1  block_type=constant  block_config=sysgen:Constant_config
  Constant5 : hdlBasic/Constant  const=0  gui_display_data_type=Boolean  arith_type=Boolean  n_bits=16  bin_pt=14  preci_type=Single  exp_width=8  frac_width=24  explicit_period=off  period=1  XmcBlockStatus=1  maskContainerNames=tabcontainer1  block_type=constant  block_config=sysgen:Constant_config
  Constant6 : hdlBasic/Constant  const=0  gui_display_data_type=Boolean  arith_type=Boolean  n_bits=16  bin_pt=13  preci_type=Single  exp_width=8  frac_width=24  explicit_period=off  period=1  XmcBlockStatus=1  maskContainerNames=tabcontainer1  block_type=constant  block_config=sysgen:Constant_config
  Constant7 : hdlBasic/Constant  const=0.0  gui_display_data_type=Fixed-point  arith_type=Signed (2's comp)  n_bits=16  bin_pt=0  preci_type=Single  exp_width=8  frac_width=24  explicit_period=off  period=1  XmcBlockStatus=1  maskContainerNames=tabcontainer1  block_type=constant  block_config=sysgen:Constant_config
  Delay1 : hdlBasic/Delay  rst=off  en=off  latency=42  reg_retiming=off  XmcBlockStatus=1  maskContainerNames=group1  block_type=delay  block_config=sysgen:Delay_config
  Delay13 : hdlBasic/Delay  rst=off  en=off  latency=42  reg_retiming=off  XmcBlockStatus=1  maskContainerNames=group1  block_type=delay  block_config=sysgen:Delay_config
  Delay2 : hdlBasic/Delay  rst=off  en=off  latency=42  reg_retiming=off  XmcBlockStatus=1  maskContainerNames=group1  block_type=delay  block_config=sysgen:Delay_config
  Mult : hdlBasic/Mult  precision=User Defined  arith_type="Signed  (2's comp)"  n_bits=16  bin_pt=13  quantization="Round  (unbiased: +/- Inf)"  overflow=Saturate  en=off  latency=0  use_behavioral_HDL=off  opt=Speed  use_embedded=on  optimum_pipeline=off  pipeline=on  use_rpm=on  placement_style=Triangular  XmcBlockStatus=1  maskContainerNames=group1  block_type=mult  block_config=sysgen:Mult_config
  Mux1 : hdlBasic/Mux  inputs=2  en=off  latency=0  precision=User Defined  arith_type="Signed  (2's comp)"  n_bits=16  bin_pt=13  quantization="Round  (unbiased: +/- Inf)"  overflow=Saturate  XmcBlockStatus=1  maskContainerNames=tabcontainer1  block_type=mux  block_config=sysgen:Mux_config
  Mux2 : hdlBasic/Mux  inputs=2  en=off  latency=0  precision=User Defined  arith_type="Signed  (2's comp)"  n_bits=16  bin_pt=13  quantization="Round  (unbiased: +/- Inf)"  overflow=Saturate  XmcBlockStatus=1  maskContainerNames=tabcontainer1  block_type=mux  block_config=sysgen:Mux_config
  Negate11 : hdlBasic/Negate  precision=User Defined  arith_type="Signed  (2's comp)"  n_bits=16  bin_pt=13  quantization=Truncate  overflow=Wrap  en=off  latency=0  XmcBlockStatus=1  maskContainerNames=tabcontainer1  block_type=negate  block_config=sysgen:Negate_config
  Scope{1..7} (7 alike) : Scope
  Terminator{1..3,5..6,8..11} (9 alike) : Terminator
  Vitis HLS2 : hdlBasic/Vitis HLS  anytable='..\Vitis_HLS\project6_final_hls_mc\solution2_add_back_substitution'  fast_sim=off  display_datatype=off  rate_propagation_method=Simulink system period  model_file_path=''  latency=1  block_type=vitis_hls
      settings: infoedit=This block allows including C,C++ and SystemC source files in System Generator for DSP designs.
  X_out : Outport
  rst_out : Outport  Port=2
  wires:
  Constant4/1 -> Vitis HLS2/2
  Vitis HLS2/4 -> Terminator10/1
  Constant2/1 -> Vitis HLS2/5
  Constant3/1 -> Vitis HLS2/6
  Constant5/1 -> Vitis HLS2/1
  Vitis HLS2/2 -> Terminator1/1
  Vitis HLS2/8 -> Terminator8/1
  Vitis HLS2/9 -> Terminator9/1
  Vitis HLS2/1 -> Terminator3/1
  Constant1/1 -> Vitis HLS2/4
  Constant6/1 -> Vitis HLS2/3
  Constant7/1 -> Vitis HLS2/7
  Vitis HLS2/3 -> Terminator2/1
  Vitis HLS2/5 -> Terminator5/1
  Vitis HLS2/7 -> Terminator6/1
  Vitis HLS2/6 -> Terminator11/1
  QTb_in/1 -> AddSub/1
  R_in/1 -> Delay13/1, Scope2/1, Mult/1
  x_in/1 -> Scope3/1, Mux1/2, Mult/2
  Mult/1 -> AddSub/2, Scope1/1
  AddSub/1 -> Scope4/1, Vitis HLS2/9
  Delay13/1 -> Vitis HLS2/8, Scope5/1
  Mux2/1 -> Negate11/1, Scope6/1
  Constant8/1 -> Mux2/2
  Vitis HLS2/10 -> Mux2/3
  Vitis HLS2/11 -> Mux2/1
  rst_in/1 -> Delay1/1
  Delay1/1 -> Delay2/1
  Delay2/1 -> rst_out/1, Mux1/1
  Mux1/1 -> X_out/1, Scope7/1
  Negate11/1 -> Mux1/3
